simulink library "usask_hyd_lib"  (R2015a)
settings: Solver=ode45  StartTime=0.0  StopTime=10.0  RelTol=1e-3
libraries: fl_lib x23, usask_hyd_ssc_lib x6, nesl_utility x4, pipeline_lib x3, usask_hyd_lib x1
settings Model: Creator=tkw954  LastModifiedBy=tkw954
settings DebuggingCC: UnderspecifiedInitializationDetection=Classic  MergeDetectMultiDrivingBlocksExec=none  SolverPrmCheckMsg=warning  StateNameClashWarn=warning

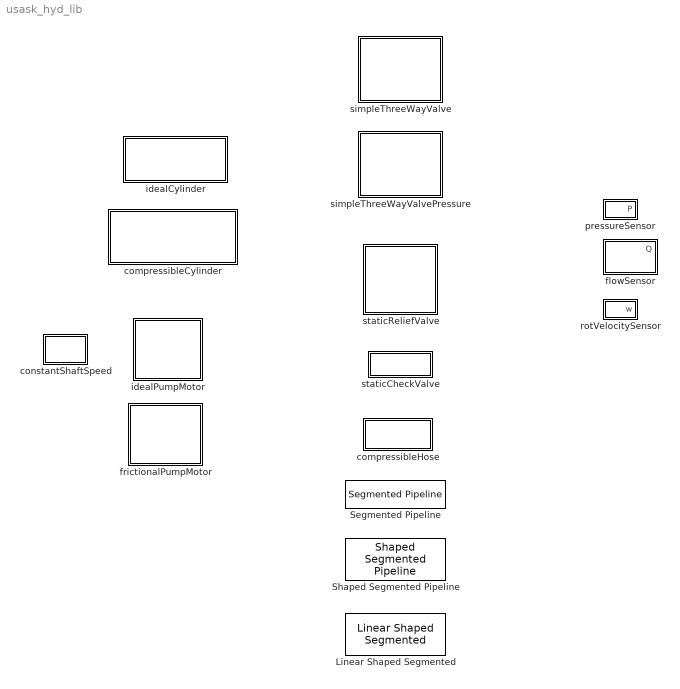
== system usask_hyd_lib ==
  Linear Shaped Segmented : pipeline_lib/Linear Shaped Segmented  N=30  x_LU=[0 1.6 2 2.5 3]  d_LU=1e-3*[10 10 20 10 10]  P0=0  Q0=0
  Segmented Pipeline : pipeline_lib/Segmented Pipeline  N=5  L=1  d=10e-3  e=1e-6  P0=0  Q0=0
  Shaped Segmented Pipeline : pipeline_lib/Shaped Segmented Pipeline  N=30  x_LU=[0 1.6 2 2.5 3]  d_LU=1e-3*[10 10 20 10 10]  e=1e-6  P0=0  Q0=0
  compressibleCylinder : Subsystem  mask{A_A=pi/4*100e-3^2, A_B=pi/4*(100e-3^2-50e-3^2), x_min=1, dx_max=0.5, x0=1.25, VA0=10e-6, VB0=10e-6, PA0=0, PB0=0, K=3e8, B=1e7}
      mask prompts: A_A "Piston Area A (m^2)"; A_B "Piston Area B (m^2)"; x_min "Closed Length (m)"; dx_max "Stroke (m)"; x0 "Initial Length (m)"; VA0 "Dead Volume A (m^3)"; VB0 "Dead Volume B (m^3)"; PA0 "Initial Pressure A (Pa)"; PB0 "Initial Pressure B (Pa)"; K "Contact Stiffness (N/m)"; B "Contact Damping (N/(m/s))"
      mask Display:
      | image('cylinder.png')
      | color('red')
      | port_label('lconn',2,'A')
      | port_label('lconn',1,'C')
      | 
      | port_label('rconn',2,'B')
      | port_label('rconn',1,'R')
  compressibleHose : Subsystem  mask(Compressible Hose){d=12e-3, L=2, dd_dP=1.2e-12, P0=0, e=0}
      mask prompts: d "Internal diameter (m)"; L "Length (m)"; dd_dP "Static pressure-diameter coefficient (m/Pa)"; P0 "Initial pressure (Pa)"; e "Internal surface roughness (m)"
      mask help:
      | Model of a circular hose with resistance and compliant wall. No inertial effects included.
      |
      | Compressible volume is lumped at port A.
      mask Display:
      | color('red')
      | port_label('lconn',1,'A')
      | port_label('rconn',1,'B')
      | 
      | color('black')
      | plot([0.1 0.9],[0.5 0.5])
      | plot([0.2 0.8],[0.4 0.4])
      | plot([0.2 0.8],[0.6 0.6])
  constantShaftSpeed : Subsystem  mask(Constant Shaft Speed){w_rpm=1750}
      mask prompts: w_rpm "Shaft speed (rev/min)"
      mask help: Outputs constant shaft speed.
      mask Display:
      | color('red')
      | port_label('rconn',1,'S')
  flowSensor : Subsystem  mask(Flow Sensor){unitNum=L/min}
      mask prompts: unitNum "Units"
      mask help: Measures flow, with positive flow from A to B.
      mask init:
      | unitScales=[1; 60000; 15850.32];
      | unitScale=unitScales(unitNum);
      mask TypeOptions unitNum: m^3/s | L/min | US gal/min
      mask Display:
      | color('red')
      | port_label('lconn',1,'A')
      | port_label('output',1,'P')
      | port_label('rconn',1,'B')
  frictionalPumpMotor : Subsystem  mask(Ideal Pump or Motor){D=200e-6, T_br=25, T_c=20, B_f=0.001, trans_coef=10, V_thresh=1e-4}
      mask prompts: D "Displacement (m^3/rev)"; T_br "Breakaway Friction Torque (Nm)"; T_c "Coulomb Friction Torque (Nm)"; B_f "Viscous friction coefficient (Nm/(rad/s))"; trans_coef "Transition Approximation Coefficient (s/rad)"; V_thresh "Linear Region Velocity Threshold (rad/s)"
      mask help:
      | This implements an ideal pump or motor with friction.  Ports A and B are hydraulic ports, port S is the shaft. Flow into port A tends to produce positive rotation on port S.
      |
      | This model includes no leakage, and assumes incompressible flow.  See "Rotational Friction" block for help with friction settings.
      mask Display:
      | image('pumpMotor.png')
      | 
      | color('red')
      | port_label('lconn',1,'S')
      | port_label('rconn',1,'A')
      | port_label('rconn',2,'B')
  idealCylinder : Subsystem  mask{A_A=pi/4*100e-3^2, A_B=pi/4*(100e-3^2-50e-3^2), x_min=1, dx_max=0.5, x0=1.25, K=3e8, B=1e7}
      mask prompts: A_A "Piston Area A (m^2)"; A_B "Piston Area B (m^2)"; x_min "Closed Length (m)"; dx_max "Stroke (m)"; x0 "Initial Length (m)"; K "Contact Stiffness (N/m)"; B "Contact Damping (N/(m/s))"
      mask Display:
      | image('cylinder.png')
      | color('red')
      | port_label('lconn',2,'A')
      | port_label('lconn',1,'C')
      | 
      | port_label('rconn',2,'B')
      | port_label('rconn',1,'R')
  idealPumpMotor : Subsystem  mask(Ideal Pump or Motor){D=200e-6}
      mask prompts: D "Displacement (m^3/rev)"
      mask help:
      | This implements an ideal pump or motor.  Ports A and B are hydraulic ports, port S is the shaft. Flow into port A tends to produce positive rotation on port S.
      |
      | This model includes no friction or leakage, and assumes incompressible flow.
      mask Display:
      | image('pumpMotor.png')
      | 
      | color('red')
      | port_label('lconn',1,'S')
      | port_label('rconn',1,'A')
      | port_label('rconn',2,'B')
  pressureSensor : Subsystem  mask(Pressure Sensor){unitNum=kPa}
      mask prompts: unitNum "Units"
      mask help: Measures gauge pressure at port A.
      mask init:
      | unitScales=[1; 1e-3; 1e-6; 0.00014503773];
      | unitScale=unitScales(unitNum);
      mask TypeOptions unitNum: Pa | kPa | MPa | psi
      mask Display:
      | color('red')
      | port_label('lconn',1,'A')
      | port_label('output',1,'P')
  rotVelocitySensor : Subsystem  mask(Rotational Velocity Sensor){unitNum=rev/min}
      mask prompts: unitNum "Units"
      mask help: Measures rotational velocity at port S.
      mask init:
      | unitScales=[1; 1/(2*pi); 60/(2*pi)];
      | unitScale=unitScales(unitNum);
      mask TypeOptions unitNum: rad/s | rev/s | rev/min
      mask Display:
      | color('red')
      | port_label('lconn',1,'S')
      | port_label('output',1,'w')
  simpleThreeWayValve : Subsystem  mask(Simple Three Way Valve){A_max=50e-6, Cd=0.61, x_max=10e-3, x_OL=0, A_L=1e-9, Re_cr=9.3}
      mask prompts: A_max "Maximum Orifice Area (m^2)"; Cd "Discharge Coefficient"; x_max "Maxium Spool Displacement (m)"; x_OL "Spool Overlap (m)"; A_L "Leakage Area (m^2)"; Re_cr "Critical Reynolds Number"
      mask help:
      | Implements an infinitely variable three way valve. The orifice areas linearly vary, reaching the maximum area at the maximum spool displacement.  The valve has symmetrical areas.
      |
      | A positive spool position on port x opens the orifice between ports P and A, while a negative position connects P and B.  If there is a positive overlap, port P will be connected to both A and B at zero position.
      |
      | This version calculates flow from pressure.
      mask Display:
      | image('simpleThreeWayValve.png')
      | color('red')
      | port_label('lconn',1,'x')
      | port_label('lconn',2,'P')
      | port_label('rconn',1,'A')
      | port_label('rconn',2,'B')
  simpleThreeWayValvePressure : Subsystem  mask(Simple Three Way Valve){A_max=50e-6, Cd=0.61, x_max=10e-3, x_OL=0, A_L=1e-9}
      mask prompts: A_max "Maximum Orifice Area (m^2)"; Cd "Discharge Coefficient"; x_max "Maxium Spool Displacement (m)"; x_OL "Spool Overlap (m)"; A_L "Leakage Area (m^2)"
      mask help:
      | Implements an infinitely variable three way valve. The orifice areas linearly vary, reaching the maximum area at the maximum spool displacement.  The valve has symmetrical areas.
      |
      | A positive spool position on port x opens the orifice between ports P and A, while a negative position connects P and B.  If there is a positive overlap, port P will be connected to both A and B at zero position.
      |
      | This version calculates pressure from flow.
      mask Display:
      | image('simpleThreeWayValve.png')
      | color('red')
      | port_label('lconn',1,'x')
      | port_label('lconn',2,'P')
      | port_label('rconn',1,'A')
      | port_label('rconn',2,'B')
  staticCheckValve : Subsystem  mask(Static Check Valve){P_cr=1e3, P_or=1e3, A_max=20e-6, A_leak=1e-9, Cd=0.61, Re_cr=9.3}
      mask prompts: P_cr "Cracking Pressure (Pa)"; P_or "Pressure Override (Pa)"; A_max "Maximum Orifice Area (m^2)"; A_leak "Leakage Area (m^2)"; Cd "Discharge Coefficient"; Re_cr "Critical Reynolds Number"
      mask help: Check valve with no dynamics. All flows are assumed to be turbulent.
      mask init:
      | if A_leak<=0
      |     error('Leakage Area must be positive')
      | end
      mask Display:
      | image('checkValve.png')
      | color('red')
      | port_label('lconn',1,'A')
      | port_label('rconn',1,'B')
  staticReliefValve : Subsystem  mask(Static Relief Valve){P_cr=10e6, P_or=1e6, A_max=20e-6, A_leak=1e-9, Cd=0.61, Re_cr=9.3}
      mask prompts: P_cr "Cracking Pressure (Pa)"; P_or "Pressure Override (Pa)"; A_max "Maximum Orifice Area (m^2)"; A_leak "Leakage Area (m^2)"; Cd "Discharge Coefficient"; Re_cr "Critical Reynolds Number"
      mask help: Relief valve with no dynamics. All flows are assumed to be turbulent.
      mask init:
      | if A_leak<=0
      |     error('Leakage Area must be positive')
      | end
      mask Display:
      | image('relief.png')
      | color('red')
      | port_label('lconn',1,'A')
      | port_label('rconn',1,'B')

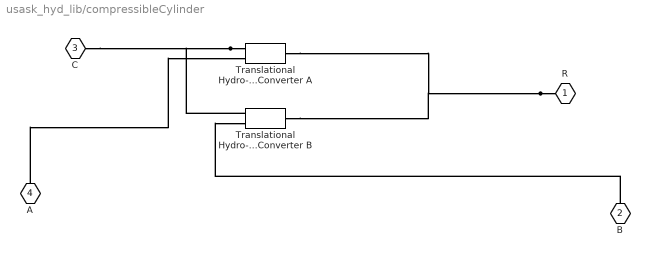
== system usask_hyd_lib/compressibleCylinder ==
  Translational Hydro-Mechanical Converter A : fl_lib/Hydraulic/Hydraulic Elements/Translational Hydro-Mechanical Converter  area=A_A m^2  or=2  compressibility=1  init_pos=x0 m  V_dead=VA0 m^3  k_sh=1.4  initial_pressure=PA0 Pa
  Translational Hydro-Mechanical Converter B : fl_lib/Hydraulic/Hydraulic Elements/Translational Hydro-Mechanical Converter  area=A_B m^2  or=1  compressibility=1  init_pos=x0 m  V_dead=VA0 m^3  k_sh=1.4  initial_pressure=PA0 Pa
  R : PMIOPort  Port=1  Side=Right
  B : PMIOPort  Port=2  Side=Right
  C : PMIOPort  Port=3  Side=Left
  A : PMIOPort  Port=4  Side=Left
  connections:
  B/RConn1 -- Translational Hydro-Mechanical Converter B/LConn2
  A/RConn1 -- Translational Hydro-Mechanical Converter A/LConn2
  Translational Hydro-Mechanical Converter A/LConn1 -- C/RConn1 -- Translational Hydro-Mechanical Converter B/LConn1
  R/RConn1 -- Translational Hydro-Mechanical Converter A/RConn1 -- Translational Hydro-Mechanical Converter B/RConn1

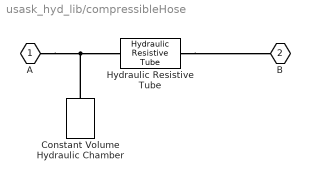
== system usask_hyd_lib/compressibleHose ==
  Constant Volume Hydraulic Chamber : fl_lib/Hydraulic/Hydraulic Elements/Constant Volume Hydraulic Chamber  ch_sp=2  wall_type=2  ch_volume=1e-4 m^3  d_in=d m  length=L m  pr_r_coef=dd_dP m/Pa  time_const=0.01 s  k_sh=1.4  p_a=101325.0 Pa  flow_rate_specify=off  flow_rate_priority=High  flow_rate=0.001 m^3/s  pressure_specify=on  pressure_priority=High  pressure=P0 Pa  diameter_incr_specify=off  diameter_incr_priority=High  diameter_incr=0 m
  Hydraulic Resistive Tube : fl_lib/Hydraulic/Hydraulic Elements/Hydraulic Resistive Tube  cs_type=1  d_in=d m  area=1e-4 m^2  D_h=1.12e-2 m  s_factor=64  length=L m  length_ad=0 m  roughness=e m  Re_lam=2000  Re_turb=4000  length_eff=6 m  rel_roughness=0.001  q_specify=off  q_priority=High  q=0.001 m^3/s  p_specify=off  p_priority=High  p=0 Pa
  A : PMIOPort  Port=1  Side=Left
  B : PMIOPort  Port=2  Side=Right
  connections:
  Hydraulic Resistive Tube/RConn1 -- B/RConn1
  Constant Volume Hydraulic Chamber/LConn1 -- A/RConn1 -- Hydraulic Resistive Tube/LConn1

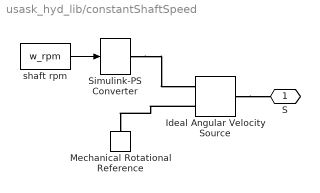
== system usask_hyd_lib/constantShaftSpeed ==
  Ideal Angular Velocity Source : fl_lib/Mechanical/Mechanical Sources/Ideal Angular Velocity Source
  Mechanical Rotational Reference : fl_lib/Mechanical/Rotational Elements/Mechanical Rotational Reference
  Simulink-PS Converter : nesl_utility/Simulink-PS Converter  PhysicalDomain=network_engine_domain  SubClassName=ps_input  LeftPortType=input  RightPortType=output  PseudoPeriodic=off  Frequencies=[]  NoiseDistribution=none  NoiseParameters=[]  Unit=rpm  AffineConversion=off  InputFiltering=off  SimscapeFilterOrder=1  InputFilterTimeConstant=0.001  UdotUserProvided=1
  shaft rpm : Constant  Value=w_rpm
  S : PMIOPort  Port=1  Side=Right
  wires:
  shaft rpm/1 -> Simulink-PS Converter/1
  connections:
  Simulink-PS Converter/RConn1 -- Ideal Angular Velocity Source/RConn1
  Ideal Angular Velocity Source/RConn2 -- Mechanical Rotational Reference/LConn1
  Ideal Angular Velocity Source/LConn1 -- S/RConn1

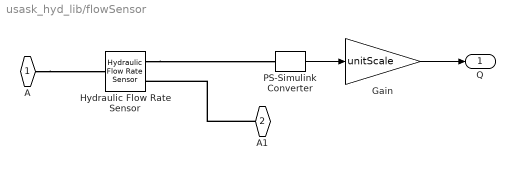
== system usask_hyd_lib/flowSensor ==
  Gain : Gain  Gain=unitScale
  Hydraulic Flow Rate Sensor : fl_lib/Hydraulic/Hydraulic Sensors/Hydraulic Flow Rate Sensor
  PS-Simulink Converter : nesl_utility/PS-Simulink Converter  PhysicalDomain=network_engine_domain  SubClassName=ps_output  LeftPortType=input  RightPortType=output  PseudoPeriodic=off  Frequencies=[]  Unit=m^3/s  AffineConversion=off
  A : PMIOPort  Port=1  Side=Left
  A1 : PMIOPort  Port=2  Side=Right
  Q : Outport
  wires:
  Gain/1 -> Q/1
  PS-Simulink Converter/1 -> Gain/1
  connections:
  A/RConn1 -- Hydraulic Flow Rate Sensor/LConn1
  Hydraulic Flow Rate Sensor/RConn1 -- PS-Simulink Converter/LConn1
  A1/RConn1 -- Hydraulic Flow Rate Sensor/RConn2

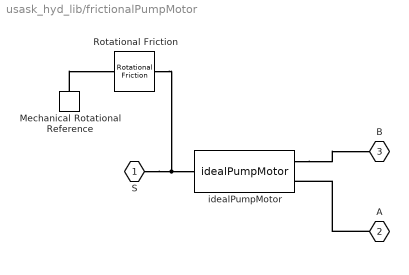
== system usask_hyd_lib/frictionalPumpMotor ==
  Mechanical Rotational Reference : fl_lib/Mechanical/Rotational Elements/Mechanical Rotational Reference
  Rotational Friction : fl_lib/Mechanical/Rotational Elements/Rotational Friction  brkwy_trq=T_br N*m  Col_trq=T_c N*m  visc_coef=B_f N*m/(rad/s)  trans_coef=trans_coef s/rad  vel_thr=V_thresh rad/s  w_specify=off  w_priority=High  w=0 rad/s  t_specify=off  t_priority=High  t=0 N*m
  idealPumpMotor : usask_hyd_lib/idealPumpMotor  D=D
  S : PMIOPort  Port=1  Side=Left
  A : PMIOPort  Port=2  Side=Right
  B : PMIOPort  Port=3  Side=Right
  connections:
  idealPumpMotor/RConn2 -- B/RConn1
  A/RConn1 -- idealPumpMotor/RConn1
  S/RConn1 -- Rotational Friction/LConn1 -- idealPumpMotor/LConn1
  Mechanical Rotational Reference/LConn1 -- Rotational Friction/RConn1

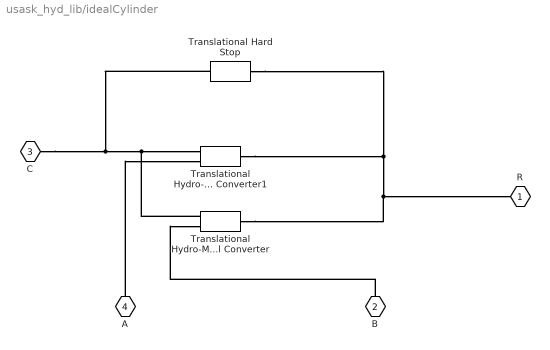
== system usask_hyd_lib/idealCylinder ==
  Translational Hydro-Mechanical Converter : fl_lib/Hydraulic/Hydraulic Elements/Translational Hydro-Mechanical Converter  area=A_B m^2  or=1  compressibility=0  init_pos=0 m  V_dead=1e-4 m^3  k_sh=1.4  initial_pressure=0 Pa
  Translational Hydro-Mechanical Converter1 : fl_lib/Hydraulic/Hydraulic Elements/Translational Hydro-Mechanical Converter  area=A_A m^2  or=2  compressibility=0  init_pos=0 m  V_dead=1e-4 m^3  k_sh=1.4  initial_pressure=0 Pa
  Translational Hard Stop : fl_lib/Mechanical/Translational Elements/Translational Hard Stop  upper_bnd=x_min+dx_max m  lower_bnd=x_min m  stiff_up=K N/m  stiff_low=K N/m  D_up=B N/(m/s)  D_low=B N/(m/s)  v_specify=off  v_priority=High  v=0 m/s  f_specify=off  f_priority=High  f=0 N  x_specify=on  x_priority=High  x=x0 m
  R : PMIOPort  Port=1  Side=Right
  B : PMIOPort  Port=2  Side=Right
  C : PMIOPort  Port=3  Side=Left
  A : PMIOPort  Port=4  Side=Left
  connections:
  B/RConn1 -- Translational Hydro-Mechanical Converter/LConn2
  A/RConn1 -- Translational Hydro-Mechanical Converter1/LConn2
  Translational Hard Stop/RConn1 -- C/RConn1 -- Translational Hydro-Mechanical Converter1/LConn1 -- Translational Hydro-Mechanical Converter/LConn1
  Translational Hard Stop/LConn1 -- Translational Hydro-Mechanical Converter1/RConn1 -- R/RConn1 -- Translational Hydro-Mechanical Converter/RConn1

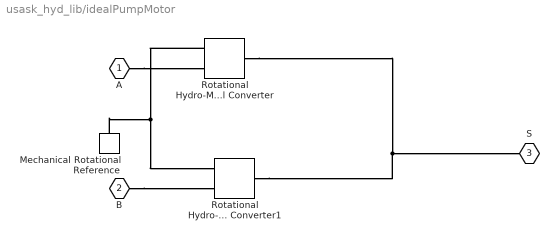
== system usask_hyd_lib/idealPumpMotor ==
  Mechanical Rotational Reference : fl_lib/Mechanical/Rotational Elements/Mechanical Rotational Reference
  Rotational Hydro-Mechanical Converter : fl_lib/Hydraulic/Hydraulic Elements/Rotational Hydro-Mechanical Converter  D=D m^3/rev  or=1  compressibility=0  initial_angle=0 rad  V_dead=1e-4 m^3  k_sh=1.4  initial_pressure=0 Pa
  Rotational Hydro-Mechanical Converter1 : fl_lib/Hydraulic/Hydraulic Elements/Rotational Hydro-Mechanical Converter  D=D m^3/rev  or=2  compressibility=0  initial_angle=0 rad  V_dead=1e-4 m^3  k_sh=1.4  initial_pressure=0 Pa
  A : PMIOPort  Port=1  Side=Right
  B : PMIOPort  Port=2  Side=Right
  S : PMIOPort  Port=3  Side=Left
  connections:
  B/RConn1 -- Rotational Hydro-Mechanical Converter1/LConn2
  A/RConn1 -- Rotational Hydro-Mechanical Converter/LConn2
  Rotational Hydro-Mechanical Converter/LConn1 -- Mechanical Rotational Reference/LConn1 -- Rotational Hydro-Mechanical Converter1/LConn1
  Rotational Hydro-Mechanical Converter1/RConn1 -- S/RConn1 -- Rotational Hydro-Mechanical Converter/RConn1

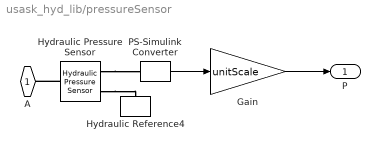
== system usask_hyd_lib/pressureSensor ==
  Gain : Gain  Gain=unitScale
  Hydraulic Pressure Sensor : fl_lib/Hydraulic/Hydraulic Sensors/Hydraulic Pressure Sensor
  Hydraulic Reference4 : fl_lib/Hydraulic/Hydraulic Elements/Hydraulic Reference
  PS-Simulink Converter : nesl_utility/PS-Simulink Converter  PhysicalDomain=network_engine_domain  SubClassName=ps_output  LeftPortType=input  RightPortType=output  PseudoPeriodic=off  Frequencies=[]  Unit=Pa  AffineConversion=off
  A : PMIOPort  Port=1  Side=Left
  P : Outport
  wires:
  PS-Simulink Converter/1 -> Gain/1
  Gain/1 -> P/1
  connections:
  Hydraulic Pressure Sensor/RConn2 -- PS-Simulink Converter/LConn1
  Hydraulic Pressure Sensor/RConn1 -- Hydraulic Reference4/LConn1
  Hydraulic Pressure Sensor/LConn1 -- A/RConn1

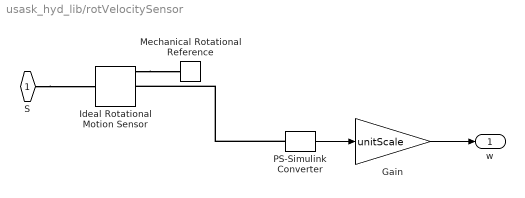
== system usask_hyd_lib/rotVelocitySensor ==
  Gain : Gain  Gain=unitScale
  Ideal Rotational Motion Sensor : fl_lib/Mechanical/Mechanical Sensors/Ideal Rotational Motion Sensor  offset=0 rad
  Mechanical Rotational Reference : fl_lib/Mechanical/Rotational Elements/Mechanical Rotational Reference
  PS-Simulink Converter : nesl_utility/PS-Simulink Converter  PhysicalDomain=network_engine_domain  SubClassName=ps_output  LeftPortType=input  RightPortType=output  PseudoPeriodic=off  Frequencies=[]  Unit=rad/s  AffineConversion=off
  S : PMIOPort  Port=1  Side=Left
  w : Outport
  wires:
  Gain/1 -> w/1
  PS-Simulink Converter/1 -> Gain/1
  connections:
  S/RConn1 -- Ideal Rotational Motion Sensor/LConn1
  PS-Simulink Converter/LConn1 -- Ideal Rotational Motion Sensor/RConn2
  Ideal Rotational Motion Sensor/RConn1 -- Mechanical Rotational Reference/LConn1

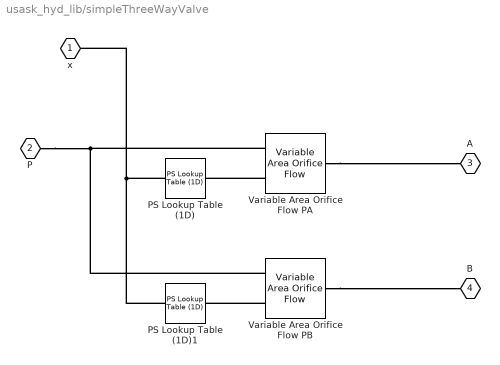
== system usask_hyd_lib/simpleThreeWayValve ==
  PS Lookup Table (1D) : fl_lib/Physical Signals/Lookup Tables/PS Lookup Table (1D)  x_t=[-x_OL x_max]  y_t=[0 A_max]  interp_method=1  extrap_method=2
  PS Lookup Table (1D)1 : fl_lib/Physical Signals/Lookup Tables/PS Lookup Table (1D)  x_t=[-x_max x_OL]  y_t=[A_max 0]  interp_method=1  extrap_method=2
  Variable Area Orifice Flow PA : usask_hyd_ssc_lib/Variable Area Orifice Flow  Cd=Cd  Al=A_L m^2  Re_cr=Re_cr  q_specify=off  q_priority=High  q=1 m^3/s  p_specify=off  p_priority=High  p=0 Pa  Pw_specify=off  Pw_priority=High  Pw=0 W
  Variable Area Orifice Flow PB : usask_hyd_ssc_lib/Variable Area Orifice Flow  Cd=Cd  Al=A_L m^2  Re_cr=Re_cr  q_specify=off  q_priority=High  q=1 m^3/s  p_specify=off  p_priority=High  p=0 Pa  Pw_specify=off  Pw_priority=High  Pw=0 W
  x : PMIOPort  Port=1  Side=Left
  P : PMIOPort  Port=2  Side=Left
  A : PMIOPort  Port=3  Side=Right
  B : PMIOPort  Port=4  Side=Right
  connections:
  P/RConn1 -- Variable Area Orifice Flow PB/LConn1 -- Variable Area Orifice Flow PA/LConn1
  Variable Area Orifice Flow PA/RConn1 -- A/RConn1
  Variable Area Orifice Flow PB/RConn1 -- B/RConn1
  Variable Area Orifice Flow PA/LConn2 -- PS Lookup Table (1D)/RConn1
  Variable Area Orifice Flow PB/LConn2 -- PS Lookup Table (1D)1/RConn1
  PS Lookup Table (1D)/LConn1 -- x/RConn1 -- PS Lookup Table (1D)1/LConn1

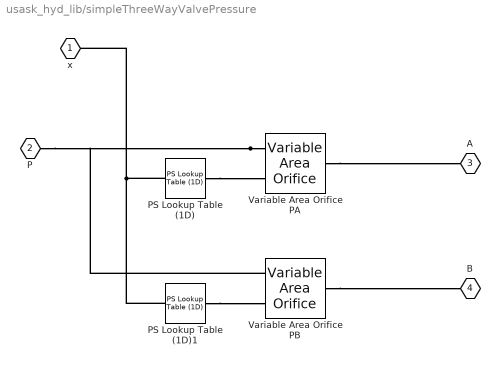
== system usask_hyd_lib/simpleThreeWayValvePressure ==
  PS Lookup Table (1D) : fl_lib/Physical Signals/Lookup Tables/PS Lookup Table (1D)  x_t=[-x_OL x_max]  y_t=[0 A_max]  interp_method=1  extrap_method=2
  PS Lookup Table (1D)1 : fl_lib/Physical Signals/Lookup Tables/PS Lookup Table (1D)  x_t=[-x_max x_OL]  y_t=[A_max 0]  interp_method=1  extrap_method=2
  Variable Area Orifice PA : usask_hyd_ssc_lib/Variable Area Orifice  Cd=Cd  Al=A_L m^2  q_specify=off  q_priority=High  q=1 m^3/s  p_specify=off  p_priority=High  p=0 Pa  Pw_specify=off  Pw_priority=High  Pw=0 W
  Variable Area Orifice PB : usask_hyd_ssc_lib/Variable Area Orifice  Cd=Cd  Al=A_L m^2  q_specify=off  q_priority=High  q=1 m^3/s  p_specify=off  p_priority=High  p=0 Pa  Pw_specify=off  Pw_priority=High  Pw=0 W
  x : PMIOPort  Port=1  Side=Left
  P : PMIOPort  Port=2  Side=Left
  A : PMIOPort  Port=3  Side=Right
  B : PMIOPort  Port=4  Side=Right
  connections:
  PS Lookup Table (1D)1/LConn1 -- x/RConn1 -- PS Lookup Table (1D)/LConn1
  PS Lookup Table (1D)1/RConn1 -- Variable Area Orifice PB/LConn2
  PS Lookup Table (1D)/RConn1 -- Variable Area Orifice PA/LConn2
  Variable Area Orifice PB/RConn1 -- B/RConn1
  Variable Area Orifice PA/RConn1 -- A/RConn1
  Variable Area Orifice PA/LConn1 -- P/RConn1 -- Variable Area Orifice PB/LConn1

== system usask_hyd_lib/staticCheckValve ==
  Check Valve : usask_hyd_ssc_lib/Check Valve  Pcr=P_cr Pa  dPor=P_or Pa  Amax=A_max m^2  Al=A_leak m^2  Cd=Cd  Re_cr=Re_cr  q_specify=off  q_priority=High  q=1 m^3/s  p_specify=off  p_priority=High  p=0 Pa  Pw_specify=off  Pw_priority=High  Pw=0 W
  A : PMIOPort  Port=1  Side=Left
  B : PMIOPort  Port=2  Side=Right
  connections:
  Check Valve/LConn1 -- A/RConn1
  Check Valve/RConn1 -- B/RConn1

== system usask_hyd_lib/staticReliefValve ==
  Check Valve : usask_hyd_ssc_lib/Check Valve  Pcr=P_cr Pa  dPor=P_or Pa  Amax=A_max m^2  Al=A_leak m^2  Cd=Cd  Re_cr=Re_cr  q_specify=off  q_priority=High  q=1 m^3/s  p_specify=off  p_priority=High  p=0 Pa  Pw_specify=off  Pw_priority=High  Pw=0 W
  A : PMIOPort  Port=1  Side=Left
  B : PMIOPort  Port=2  Side=Right
  connections:
  Check Valve/RConn1 -- B/RConn1
  Check Valve/LConn1 -- A/RConn1
